simulink model "InteractiveArmModel_R2021a_v1"  (R2021a)
settings: Solver=ode4  StartTime=0.0  StopTime=3000  FixedStep=1/150  MaxStep=1/50  MinStep=1/200  RelTol=1e-5  AbsTol=1e-6  EnableMultiTasking=on
model workspace (MAT data in the model file):
  MaxEccentricFlexor = 0.5
  PoleZ = 0.85
  SampleTime = 0.05
  musNoise = 0
  musNoiseLevel : Simulink.Parameter (value not decoded)
libraries: simulink x1
(part 3 of 3)

== system InteractiveArmModel_R2021a_v1/Trial Start//Stop//Increment Control/Flag for What Phase Trial is In/If Action Subsystem6 ==
  In1 : Inport
  Action Port : ActionPort  ActionPortLabel=elseif(u2 == 0)
  Out1 : Outport
  wires:
  In1/1 -> Out1/1

== system InteractiveArmModel_R2021a_v1/Trial Start//Stop//Increment Control/Flag for What Phase Trial is In/If Action Subsystem7 ==
  In1 : Inport
  Action Port : ActionPort  ActionPortLabel=else
  Out1 : Outport
  wires:
  In1/1 -> Out1/1

== system InteractiveArmModel_R2021a_v1/Trial Start//Stop//Increment Control/Stop Criteria Flag Control (Between Trials)/If Action Subsystem3 ==
  In1 : Inport
  Action Port : ActionPort  ActionPortLabel=if(u1 == 0)
  Out1 : Outport
  wires:
  In1/1 -> Out1/1

== system InteractiveArmModel_R2021a_v1/Trial Start//Stop//Increment Control/Stop Criteria Flag Control (Between Trials)/If Action Subsystem4 ==
  In1 : Inport
  Action Port : ActionPort  ActionPortLabel=else
  Out1 : Outport
  wires:
  In1/1 -> Out1/1

== system InteractiveArmModel_R2021a_v1/Trial Start//Stop//Increment Control/Subsystem/If Action Subsystem ==
  In1 : Inport
  Action Port : ActionPort  ActionPortLabel=if(u1 == 0)
  Out1 : Outport
  wires:
  In1/1 -> Out1/1

== system InteractiveArmModel_R2021a_v1/Trial Start//Stop//Increment Control/Subsystem2/If Action Subsystem1 ==
  In1 : Inport
  Action Port : ActionPort  ActionPortLabel=if(u1 < 0.01)
  Out1 : Outport
  wires:
  In1/1 -> Out1/1

== system InteractiveArmModel_R2021a_v1/Trial Start//Stop//Increment Control/Subsystem2/If Action Subsystem2 ==
  In1 : Inport
  Action Port : ActionPort  ActionPortLabel=else
  Out1 : Outport
  wires:
  In1/1 -> Out1/1

== system InteractiveArmModel_R2021a_v1/While Loop (Main Simulation Code)/Integrator 1/Integrater ==
  Accel : Inport
  Add : Sum
  Delay : Delay  DelayLength=1  InitialCondition=0
  Delay1 : Delay  DelayLength=1  InitialCondition=0
  Digital Clock : DigitalClock  SampleTime=-1
  Product : Product
  Subtract : Sum  Inputs=+-
  Vel : Outport
  wires:
  Accel/1 -> Product/2
  Subtract/1 -> Product/1
  Product/1 -> Add/1
  Add/1 -> Delay/1
  Delay/1 -> Vel/1, Add/2
  Digital Clock/1 -> Subtract/1, Delay1/1
  Delay1/1 -> Subtract/2

== system InteractiveArmModel_R2021a_v1/While Loop (Main Simulation Code)/Integrator 1/Reset ==
  Reset : Inport
  " Accel" : Inport  Port=2
  If : If  IfExpression=u1 == 0  ShowElse=off
  If Action Subsystem : Subsystem  TreatAsAtomicUnit=on
  Subtract : Sum  Inputs=+-
  Accel : Outport
  wires:
  Reset/1 -> If/1
  If/1 -> If Action Subsystem/Action
  Subtract/1 -> Accel/1
  " Accel"/1 -> Subtract/1, If Action Subsystem/1(In1)
  If Action Subsystem/1(Out1) -> Subtract/2

== system InteractiveArmModel_R2021a_v1/While Loop (Main Simulation Code)/Integrator 1/Reset2 ==
  Reset : Inport
  VelIn : Inport  Port=2
  If : If  IfExpression=u1 == 0  ShowElse=off
  If Action Subsystem : Subsystem  TreatAsAtomicUnit=on
  Subtract : Sum  Inputs=+-
  VelOut : Outport
  wires:
  Reset/1 -> If/1
  If/1 -> If Action Subsystem/Action
  Subtract/1 -> VelOut/1
  VelIn/1 -> Subtract/1, If Action Subsystem/1(In1)
  If Action Subsystem/1(Out1) -> Subtract/2

== system InteractiveArmModel_R2021a_v1/While Loop (Main Simulation Code)/Integrator 2/Integrater 1 ==
  VelIn : Inport
  Add : Sum
  Delay : Delay  DelayLength=1  InitialCondition=0
  Delay1 : Delay  DelayLength=1  InitialCondition=0
  Digital Clock : DigitalClock  SampleTime=-1
  Product : Product
  Subtract : Sum  Inputs=+-
  PosOut : Outport
  wires:
  VelIn/1 -> Product/2
  Subtract/1 -> Product/1
  Product/1 -> Add/1
  Add/1 -> Delay/1
  Delay/1 -> PosOut/1, Add/2
  Digital Clock/1 -> Subtract/1, Delay1/1
  Delay1/1 -> Subtract/2

== system InteractiveArmModel_R2021a_v1/While Loop (Main Simulation Code)/Integrator 2/Reset2 ==
  Reset : Inport
  PosIn : Inport  Port=2
  If : If  IfExpression=u1 == 0  ShowElse=off
  If Action Subsystem : Subsystem  TreatAsAtomicUnit=on
  Subtract : Sum  Inputs=+-
  PosOut : Outport
  wires:
  Reset/1 -> If/1
  If/1 -> If Action Subsystem/Action
  Subtract/1 -> PosOut/1
  PosIn/1 -> Subtract/1, If Action Subsystem/1(In1)
  If Action Subsystem/1(Out1) -> Subtract/2

== system InteractiveArmModel_R2021a_v1/While Loop (Main Simulation Code)/Muscle Models/Add Noise to Keyboard // Mouse Control Input Types ==
  In1 : Inport
  Add1 : Sum
  Add2 : Sum
  Demux2 : Demux  Outputs=2
  If : If  IfExpression=u1 > 0.01
  If Action Subsystem : Subsystem  TreatAsAtomicUnit=on
  If Action Subsystem1 : Subsystem  TreatAsAtomicUnit=on
  If Action Subsystem2 : Subsystem  TreatAsAtomicUnit=on
  If Action Subsystem3 : Subsystem  TreatAsAtomicUnit=on
  If2 : If  IfExpression=u1 > 0.01
  Merge : Merge
  Merge2 : Merge
  Mux1 : Mux  Inputs=2
  Random Number : RandomNumber  Variance=musNoise
  Random Number1 : RandomNumber  Variance=musNoise
  Scope : Scope
  Out1 : Outport
  wires:
  If Action Subsystem2/1(Out1) -> Merge2/1
  If/2 -> If Action Subsystem1/Action
  Demux2/1 -> If/1, If Action Subsystem1/1(In1), Add1/1
  Random Number/1 -> Scope/1, Add1/2
  Demux2/2 -> If2/1, Add2/1, If Action Subsystem3/1(In1)
  Merge/1 -> Mux1/1
  Add1/1 -> If Action Subsystem/1(In1)
  Merge2/1 -> Mux1/2
  Add2/1 -> If Action Subsystem2/1(In1)
  If Action Subsystem3/1(Out1) -> Merge2/2
  If2/2 -> If Action Subsystem3/Action
  If2/1 -> If Action Subsystem2/Action
  If Action Subsystem1/1(Out1) -> Merge/2
  Random Number1/1 -> Add2/2
  If/1 -> If Action Subsystem/Action
  If Action Subsystem/1(Out1) -> Merge/1
  In1/1 -> Demux2/1
  Mux1/1 -> Out1/1

== system InteractiveArmModel_R2021a_v1/While Loop (Main Simulation Code)/Muscle Models/EMG Calibration1 ==
  stimulation(flex+Ext) : Inport
  Demux : Demux  Outputs=2
  Divide : Product  Inputs=*/
  Divide1 : Product  Inputs=*/
  Maxima Ext : Constant  Value=980
  Maxima Flex : Constant  Value=980
  Minima Ext : Constant  Value=80
  Minima Flex : Constant  Value=50
  Mux : Mux  Inputs=2
  Saturation : Saturate  UpperLimit=1  LowerLimit=0
  Saturation1 : Saturate  UpperLimit=1  LowerLimit=0
  Subtract{1..4} (4 alike) : Sum  Inputs=+-
  Excitation (Range: 0-1) : Outport
  wires:
  Subtract3/1 -> Divide/2
  Subtract4/1 -> Divide/1
  Divide/1 -> Saturation/1
  Minima Flex/1 -> Subtract3/2, Subtract4/2
  Maxima Flex/1 -> Subtract3/1
  stimulation(flex+Ext)/1 -> Demux/1
  Demux/1 -> Subtract4/1  "FLEX"
  Demux/2 -> Subtract2/1  "EXT"
  Saturation1/1 -> Mux/2
  Subtract2/1 -> Divide1/1
  Divide1/1 -> Saturation1/1
  Minima Ext/1 -> Subtract1/2, Subtract2/2
  Subtract1/1 -> Divide1/2
  Maxima Ext/1 -> Subtract1/1
  Mux/1 -> Excitation (Range: 0-1)/1
  Saturation/1 -> Mux/1

== system InteractiveArmModel_R2021a_v1/While Loop (Main Simulation Code)/Muscle Models/EMG Control ==
  stimulation(flex+Ext) : Inport
  Action Port : ActionPort  ActionPortLabel=elseif( u1 == 2)
  Out1 : Outport
  wires:
  stimulation(flex+Ext)/1 -> Out1/1

== system InteractiveArmModel_R2021a_v1/While Loop (Main Simulation Code)/Muscle Models/Extensor Muscle Mechanics ==
  note: Activation
  "Excitation Extensor " : Inport
  IC : Inport  Port=2
  LMT Extensor : Inport  Port=3
  ModelAge : Inport  Port=4
  Bounds Checks : Subsystem
  Constant13 : Constant
  Delay : Delay  DelayLength=1  InitialCondition=0
  Force-Velocity Relation : FunctionCaller  FunctionPrototype=[vSEE,dPdt,vCE] = Muscle_Mechanics_Functions.FVR(FP,Vmt,p,flexext,activation,ModelStrength)  InputArgumentSpecifications=<Enter example>  OutputArgumentSpecifications=<Enter example>
  Function Caller : FunctionCaller  FunctionPrototype=ActivationChange = Muscle_Mechanics_Functions.ExciteAct(IC,Excitation,WhichMus,PreviousAct)  InputArgumentSpecifications=<Enter example>  OutputArgumentSpecifications=<Enter example>
  Function Caller1 : FunctionCaller  FunctionPrototype=[FP,LCC] = Muscle_Mechanics_Functions.FLR(Lmt,L_SEE,Activation,FlexExt,ModelStrength)  InputArgumentSpecifications=<Enter example>  OutputArgumentSpecifications=<Enter example>
  Function Caller3 : FunctionCaller  FunctionPrototype=L_SEE = Muscle_Mechanics_Functions.LSEE(P,FlexOrExtMus,ModelStrength)  InputArgumentSpecifications=<Enter example>  OutputArgumentSpecifications=<Enter example>
  IEEE Double Discrete Time Filtered Derivative : DiscreteFilter  Numerator=(1-PoleZ)*[1 -1]  Denominator=SampleTime*[1 -PoleZ]
  Integrate Act Change : Subsystem
  Reset : Subsystem
  Subsystem : Subsystem
  To Workspace1 : ToWorkspace  VariableName=activationExt  SaveFormat=Timeseries  SampleTime=-1
  To Workspace2 : ToWorkspace  VariableName=forcePotentialExt  SaveFormat=Timeseries  SampleTime=-1
  To Workspace3 : ToWorkspace  VariableName=lengthCC_Ext  SaveFormat=Timeseries  SampleTime=-1
  To Workspace4 : ToWorkspace  VariableName=musVelExt  SaveFormat=Timeseries  SampleTime=-1
  To Workspace5 : ToWorkspace  VariableName=velSEE_Ext  SaveFormat=Timeseries  SampleTime=-1
  To Workspace6 : ToWorkspace  VariableName=lenSEE_Ext  SaveFormat=Timeseries  SampleTime=-1
  To Workspace7 : ToWorkspace  VariableName=musLenExt  SaveFormat=Timeseries  SampleTime=-1
  To Workspace8 : ToWorkspace  VariableName=velCE_Ext  SaveFormat=Timeseries  SampleTime=-1
  P Extenasor : Outport
  wires:
  Constant13/1 -> Function Caller3/2, Function Caller1/4, Force-Velocity Relation/4, Function Caller/3
  Function Caller3/1 -> To Workspace6/1, Function Caller1/2  "Ext LSEE"
  Function Caller1/1 -> To Workspace2/1, Force-Velocity Relation/1  "Ext FP"
  Function Caller1/2 -> To Workspace3/1  "Ext LCC"
  LMT Extensor/1 -> IEEE Double Discrete Time Filtered Derivative/1, To Workspace7/1, Function Caller1/1  "Lmt"
  Subsystem/1(Force) -> Reset/2(" ")  "P Extenasor"
  Reset/1("Force ") -> Bounds Checks/2("Force ")
  Force-Velocity Relation/2 -> Subsystem/1(dp/dt)
  Force-Velocity Relation/1 -> To Workspace5/1  "dP/dt Extensor"
  Force-Velocity Relation/3 -> To Workspace8/1
  "Excitation Extensor "/1 -> Function Caller/2
  Delay/1 -> Function Caller/4
  IC/1 -> Function Caller/1, Reset/1(1), Integrate Act Change/1(IC)
  Integrate Act Change/1(Activation) -> Function Caller1/3, Force-Velocity Relation/5, Delay/1, Bounds Checks/1(Activation), To Workspace1/1
  Function Caller/1 -> Integrate Act Change/2(In2)
  Bounds Checks/1(P Flexor) -> P Extenasor/1, Function Caller3/1, Force-Velocity Relation/3
  ModelAge/1 -> Bounds Checks/3(ModelAge), Force-Velocity Relation/6, Function Caller1/5, Function Caller3/3
  IEEE Double Discrete Time Filtered Derivative/1 -> Force-Velocity Relation/2, To Workspace4/1  "Discrete-Time Filtered Derivative"

== system InteractiveArmModel_R2021a_v1/While Loop (Main Simulation Code)/Muscle Models/Flexor Muscle Mechanics ==
  note: From "Fixed-Point Derivatives" simulink example.
      | https://www.mathworks.com/help/fixedpoint/ug/fixed-point-derivatives.html
  note: Activation
  ExcitationFlexor : Inport
  IC : Inport  Port=2
  LmtFlexor : Inport  Port=3
  ModelAge : Inport  Port=4
  Bounds Checks : Subsystem
  Delay : Delay  DelayLength=1  InitialCondition=0
  FlexorOrExtensorConstant : Constant  Value=2
  Force-Extension Relation : FunctionCaller  FunctionPrototype=L_SEE = Muscle_Mechanics_Functions.LSEE(P,FlexOrExtMus,ModelStrength)  InputArgumentSpecifications=<Enter example>  OutputArgumentSpecifications=<Enter example>
  Force-Length Relationship : FunctionCaller  FunctionPrototype=[FP,LCC] = Muscle_Mechanics_Functions.FLR(Lmt,L_SEE,Activation,FlexExt,ModelStrength)  InputArgumentSpecifications=<Enter example>  OutputArgumentSpecifications=<Enter example>
  Force-Velocity Relationship : FunctionCaller  FunctionPrototype=[vSEE,dPdt,vCE] = Muscle_Mechanics_Functions.FVR(FP,Vmt,p,flexext,activation,ModelStrength)  InputArgumentSpecifications=<Enter example>  OutputArgumentSpecifications=<Enter example>
  Function Caller1 : FunctionCaller  FunctionPrototype=ActivationChange = Muscle_Mechanics_Functions.ExciteAct(IC,Excitation,WhichMus,PreviousAct)  InputArgumentSpecifications=<Enter example>  OutputArgumentSpecifications=<Enter example>
  IEEE Double Discrete Time Filtered Derivative : DiscreteFilter  Numerator=(1-PoleZ)*[1 -1]  Denominator=SampleTime*[1 -PoleZ]
  Integrate Act Change : Subsystem
  Integrater : Subsystem
  Reset : Subsystem
  To Workspace10 : ToWorkspace  VariableName=velCE_Flex1  SaveFormat=Timeseries  SampleTime=-1
  To Workspace3 : ToWorkspace  VariableName=activationFlex1  SaveFormat=Timeseries  SampleTime=-1
  To Workspace4 : ToWorkspace  VariableName=forcePotentialFlex1  SaveFormat=Timeseries  SampleTime=-1
  To Workspace5 : ToWorkspace  VariableName=lengthCC_Flex1  SaveFormat=Timeseries  SampleTime=-1
  To Workspace6 : ToWorkspace  VariableName=musVelFlex1  SaveFormat=Timeseries  SampleTime=-1
  To Workspace7 : ToWorkspace  VariableName=lenSEE_Flex1  SaveFormat=Timeseries  SampleTime=-1
  To Workspace8 : ToWorkspace  VariableName=velSEE_Flex1  SaveFormat=Timeseries  SampleTime=-1
  To Workspace9 : ToWorkspace  VariableName=musLenFlex1  SaveFormat=Timeseries  SampleTime=-1
  P Flexor : Outport
  wires:
  FlexorOrExtensorConstant/1 -> Function Caller1/3, Force-Extension Relation/2, Force-Length Relationship/4, Force-Velocity Relationship/4
  IEEE Double Discrete Time Filtered Derivative/1 -> To Workspace6/1, Force-Velocity Relationship/2  "Discrete-Time Filtered Derivative"
  Force-Length Relationship/2 -> To Workspace5/1  "Flex LCC"
  Bounds Checks/1(P Flexor) -> Force-Extension Relation/1, Force-Velocity Relationship/3, P Flexor/1
  Integrater/1(1) -> Reset/2(" ")  "P Extenasor"
  Integrate Act Change/1(Out1) -> Force-Velocity Relationship/5, Delay/1, Force-Length Relationship/3, Bounds Checks/1(Activation), To Workspace3/1
  Reset/1("Force ") -> Bounds Checks/2("Force ")
  ModelAge/1 -> Bounds Checks/3(ModelAge), Force-Velocity Relationship/6, Force-Length Relationship/5, Force-Extension Relation/3
  LmtFlexor/1 -> IEEE Double Discrete Time Filtered Derivative/1, To Workspace9/1, Force-Length Relationship/1
  IC/1 -> Integrate Act Change/1(IC), Function Caller1/1, Reset/1(1)
  Force-Length Relationship/1 -> To Workspace4/1, Force-Velocity Relationship/1  "Flex FP"
  Force-Velocity Relationship/2 -> Integrater/1(In1)
  Force-Extension Relation/1 -> To Workspace7/1, Force-Length Relationship/2  "Flex LSEE"
  Force-Velocity Relationship/1 -> To Workspace8/1  "dP/dt"
  Delay/1 -> Function Caller1/4
  ExcitationFlexor/1 -> Function Caller1/2
  Function Caller1/1 -> Integrate Act Change/2(In2)
  Force-Velocity Relationship/3 -> To Workspace10/1

== system InteractiveArmModel_R2021a_v1/While Loop (Main Simulation Code)/Muscle Models/Keyboard Control ==
  stimulation(flex+Ext) : Inport
  Action Port : ActionPort  ActionPortLabel=if(u1 == 0)
  Out1 : Outport
  wires:
  stimulation(flex+Ext)/1 -> Out1/1

== system InteractiveArmModel_R2021a_v1/While Loop (Main Simulation Code)/Muscle Models/Mouse Control ==
  stimulation(flex+Ext) : Inport
  Action Port : ActionPort  ActionPortLabel=elseif(u1 == 1)
  Out1 : Outport
  wires:
  stimulation(flex+Ext)/1 -> Out1/1

== system InteractiveArmModel_R2021a_v1/While Loop (Main Simulation Code)/Musculoskeletal Geometry/LMT Extensor ==
  angle (r) : Inport
  Lower Arm length (m) : Inport  Port=2
  upper arm length (m) : Inport  Port=3
  Add : Sum
  Constant : Constant  Value=0.1
  Constant1 : Constant  Value=0.9
  Cos : Trigonometry  Operator=cos
  Math Function : Math  Operator=square  SaturateOnIntegerOverflow=on
  Math Function1 : Math  Operator=square  SaturateOnIntegerOverflow=on
  Product{1..4} (4 alike) : Product
  Sqrt : Sqrt  SaturateOnIntegerOverflow=on
  Subtract : Sum  Inputs=+-
  Trigonometric Function : Trigonometry
  Lmt Extensor (m) : Outport
  Proximal Ext Muscle attachment (m),x : Outport  Port=2
  Distal Ext Muscle Attachment (m) ,x : Outport  Port=3
  Distal Ext Muscle Attachment (m) ,y : Outport  Port=4
  wires:
  Subtract/1 -> Math Function/1
  Math Function/1 -> Add/2
  angle (r)/1 -> Trigonometric Function/1, Cos/1
  Constant1/1 -> Product1/2
  Add/1 -> Sqrt/1
  Product4/1 -> Distal Ext Muscle Attachment (m) ,y/1, Math Function1/1
  Product1/1 -> Proximal Ext Muscle attachment (m),x/1, Subtract/2
  Product3/1 -> Distal Ext Muscle Attachment (m) ,x/1, Subtract/1
  Product2/1 -> Product3/2, Product4/2
  Cos/1 -> Product3/1
  Math Function1/1 -> Add/1
  Constant/1 -> Product2/1
  upper arm length (m)/1 -> Product1/1
  Lower Arm length (m)/1 -> Product2/2
  Sqrt/1 -> Lmt Extensor (m)/1
  Trigonometric Function/1 -> Product4/1

== system InteractiveArmModel_R2021a_v1/While Loop (Main Simulation Code)/Musculoskeletal Geometry/LMT Flexor ==
  angle (r) : Inport
  lower arm length (m) : Inport  Port=2
  upper arm length (m) : Inport  Port=3
  Add : Sum
  Add1 : Sum
  Constant : Constant  Value=0.1
  Constant1 : Constant  Value=0.9
  Cos : Trigonometry  Operator=cos
  Math Function : Math  Operator=square  SaturateOnIntegerOverflow=on
  Math Function1 : Math  Operator=square  SaturateOnIntegerOverflow=on
  Product{1..4} (4 alike) : Product
  Sqrt : Sqrt  SaturateOnIntegerOverflow=on
  Trigonometric Function : Trigonometry
  Lmt Flexor (m) : Outport
  "Proximal Flex muscle Attachment (m), x " : Outport  Port=2
  "Distal Flex muscle Attachment (m), x" : Outport  Port=3
  "Distal Flex muscle Attachment (m), y " : Outport  Port=4
  wires:
  Add1/1 -> Math Function/1
  Math Function/1 -> Add/2
  angle (r)/1 -> Trigonometric Function/1, Cos/1
  Constant1/1 -> Product1/2
  Add/1 -> Sqrt/1
  Product4/1 -> "Distal Flex muscle Attachment (m), y "/1, Math Function1/1
  Product1/1 -> Add1/2, "Proximal Flex muscle Attachment (m), x "/1
  Product3/1 -> Add1/1, "Distal Flex muscle Attachment (m), x"/1
  Product2/1 -> Product4/2, Product3/2
  Cos/1 -> Product3/1
  Math Function1/1 -> Add/1
  Constant/1 -> Product2/1
  upper arm length (m)/1 -> Product1/1
  lower arm length (m)/1 -> Product2/2
  Sqrt/1 -> Lmt Flexor (m)/1
  Trigonometric Function/1 -> Product4/1

== system InteractiveArmModel_R2021a_v1/While Loop (Main Simulation Code)/Musculoskeletal Geometry/MA Extensor ==
  angle (radians) : Inport
  Lmt Extensor (m) : Inport  Port=2
  lower arm length (m) : Inport  Port=3
  Upper arm length (m) : Inport  Port=4
  Asin : Trigonometry  Operator=asin
  Constant2 : Constant  Value=-1
  Divide : Product  Inputs=*/
  Location of Muscle Insertion : FunctionCaller  FunctionPrototype=y = Constants.insertLoc()  OutputArgumentSpecifications=<Enter example>
  Location of Muscle Origin : FunctionCaller  FunctionPrototype=y = Constants.originLoc()  OutputArgumentSpecifications=<Enter example>
  Product : Product  Inputs=3
  Product1 : Product  Inputs=3
  Product2 : Product
  Trigonometric Function : Trigonometry
  Trigonometric Function1 : Trigonometry
  Extensor Moment arm (m) : Outport
  wires:
  Product1/1 -> Divide/1
  Trigonometric Function1/1 -> Product/2
  Upper arm length (m)/1 -> Product/3
  Trigonometric Function/1 -> Product1/1
  Divide/1 -> Asin/1
  lower arm length (m)/1 -> Product1/3
  Location of Muscle Insertion/1 -> Product1/2
  Asin/1 -> Trigonometric Function1/1
  Lmt Extensor (m)/1 -> Divide/2
  angle (radians)/1 -> Trigonometric Function/1
  Product/1 -> Extensor Moment arm (m)/1
  Constant2/1 -> Product2/1
  Location of Muscle Origin/1 -> Product2/2
  Product2/1 -> Product/1

== system InteractiveArmModel_R2021a_v1/While Loop (Main Simulation Code)/Musculoskeletal Geometry/MA Flexor ==
  note: The distance from the elbow to the origin of the flexors and extensors is 90% of the length of the upper arm (starting from the elbow and going proximal).
  note: The distance from the elbow to the insertion of the flexor and extensors is 10% of the length of the lower arm (starting from the elbow and going distal).
  note: Location of flexor/ext origin is 10% of distance from shoulder to elbow (going distal from shoulder).
  angle (radians) : Inport
  Lmt Extensor (m) : Inport  Port=2
  Lower arm length (m) : Inport  Port=3
  Upper arm length (m) : Inport  Port=4
  Asin : Trigonometry  Operator=asin
  Divide : Product  Inputs=*/
  Location of Muscle Insertion : FunctionCaller  FunctionPrototype=y = Constants.insertLoc()  OutputArgumentSpecifications=<Enter example>
  Location of Muscle Origin : FunctionCaller  FunctionPrototype=y = Constants.originLoc()  OutputArgumentSpecifications=<Enter example>
  Product : Product  Inputs=3
  Product1 : Product  Inputs=3
  Trigonometric Function : Trigonometry
  Trigonometric Function1 : Trigonometry
  Flexor moment arm (m) : Outport
  wires:
  Product1/1 -> Divide/1
  Trigonometric Function1/1 -> Product/2
  Upper arm length (m)/1 -> Product/3
  Trigonometric Function/1 -> Product1/1
  Divide/1 -> Asin/1
  Lower arm length (m)/1 -> Product1/3
  Asin/1 -> Trigonometric Function1/1
  Lmt Extensor (m)/1 -> Divide/2
  angle (radians)/1 -> Trigonometric Function/1
  Product/1 -> Flexor moment arm (m)/1
  Location of Muscle Origin/1 -> Product/1
  Location of Muscle Insertion/1 -> Product1/2

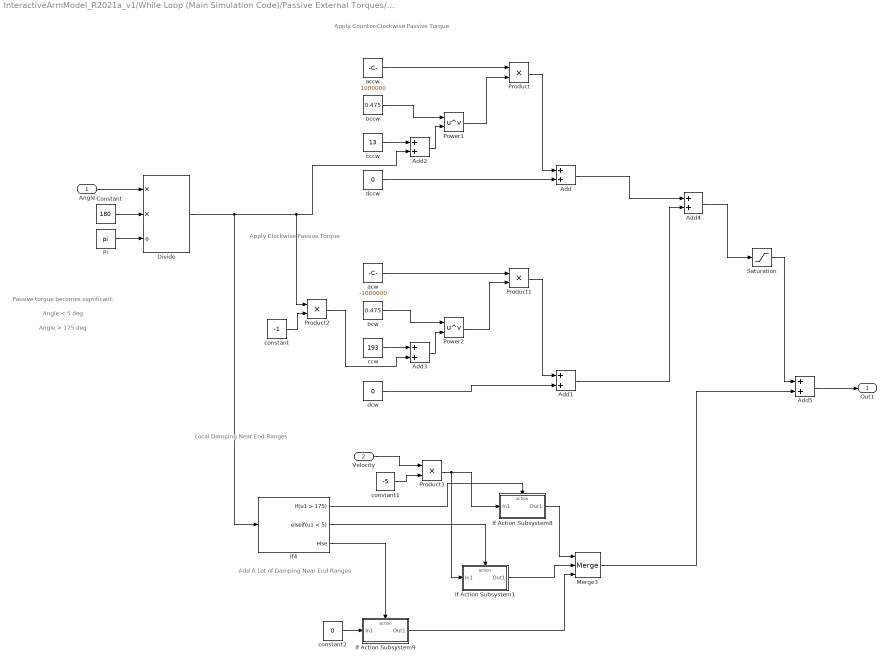
== system InteractiveArmModel_R2021a_v1/While Loop (Main Simulation Code)/Passive External Torques/Passive torque ==
  note: Apply Clockwise Passive Torque
  note: Apply Counter-Clockwise Passive Torque
  note: Local Damping Near End Ranges
  note: Add A Lot of Damping Near End Ranges
  note: Angle > 175 deg
  note: Angle < 5 deg
  note: Passive torque becomes significant:
  Angle : Inport
  Velocity : Inport  Port=2
  Add{,1..5} (6 alike) : Sum
  Constant : Constant  Value=180
  Divide : Product  Inputs=**/
  If Action Subsystem1 : Subsystem  TreatAsAtomicUnit=on
  If Action Subsystem8 : Subsystem  TreatAsAtomicUnit=on
  If Action Subsystem9 : Subsystem  TreatAsAtomicUnit=on
  If4 : If  IfExpression=u1 > 175  ElseIfExpressions=u1 < 5
  Merge3 : Merge  Inputs=3
  Pi : Constant  Value=pi  OutDataTypeStr=Inherit: Inherit via back propagation
  Power1 : Math  Operator=pow  SaturateOnIntegerOverflow=on
  Power2 : Math  Operator=pow  SaturateOnIntegerOverflow=on
  Product{,1..3} (4 alike) : Product
  Saturation : Saturate  UpperLimit=100  LowerLimit=-100
  accw : Constant  Value=1000000
  acw : Constant  Value=-1000000
  bccw : Constant  Value=0.475
  bcw : Constant  Value=0.475
  cccw : Constant  Value=13
  ccw : Constant  Value=193
  constant : Constant  Value=-1
  constant1 : Constant  Value=-5
  constant2 : Constant  Value=0
  dccw : Constant  Value=0
  dcw : Constant  Value=0
  Out1 : Outport
  wires:
  Add2/1 -> Power1/2
  Product1/1 -> Add1/1
  Power2/1 -> Product1/2
  constant/1 -> Product2/2
  Add/1 -> Add4/1
  Divide/1 -> If4/1, Product2/1, Add2/2
  accw/1 -> Product/1
  Power1/1 -> Product/2
  acw/1 -> Product1/1
  Add3/1 -> Power2/2
  bcw/1 -> Power2/1
  Product2/1 -> Add3/2
  dcw/1 -> Add1/2
  dccw/1 -> Add/2
  bccw/1 -> Power1/1
  Product/1 -> Add/1
  cccw/1 -> Add2/1
  ccw/1 -> Add3/1
  Angle/1 -> Divide/1
  Constant/1 -> Divide/2
  Pi/1 -> Divide/3
  Add1/1 -> Add4/2
  Product3/1 -> If Action Subsystem1/1(In1), If Action Subsystem8/1(In1)
  If4/1 -> If Action Subsystem8/Action
  If Action Subsystem8/1(Out1) -> Merge3/1
  If4/3 -> If Action Subsystem9/Action
  If Action Subsystem9/1(Out1) -> Merge3/3
  Velocity/1 -> Product3/1
  constant1/1 -> Product3/2
  constant2/1 -> If Action Subsystem9/1(In1)
  If4/2 -> If Action Subsystem1/Action
  If Action Subsystem1/1(Out1) -> Merge3/2
  Merge3/1 -> Add5/2
  Add5/1 -> Out1/1
  Add4/1 -> Saturation/1
  Saturation/1 -> Add5/1

== system InteractiveArmModel_R2021a_v1/Muscle_Mechanics_Functions/Contractile Element Force-Length Relation/S1, S2, S3 calculation/S1 ==
  note: C
  note: L
  In1 : Inport
  In2 : Inport  Port=2
  Constant : Constant
  Math Function : Math  Operator=square  SaturateOnIntegerOverflow=on
  Product : Product
  Subtract : Sum  Inputs=+-
  Out1 : Outport
  wires:
  In1/1 -> Math Function/1
  Math Function/1 -> Product/1
  In2/1 -> Product/2
  Product/1 -> Subtract/2
  Constant/1 -> Subtract/1
  Subtract/1 -> Out1/1

== system InteractiveArmModel_R2021a_v1/Muscle_Mechanics_Functions/Contractile Element Force-Length Relation/S1, S2, S3 calculation/S2 ==
  note: C
  note: L
  In1 : Inport
  In2 : Inport  Port=2
  In3 : Inport  Port=3
  Constant : Constant  Value=-2
  Divide : Product  Inputs=*/
  Exp : Math  SaturateOnIntegerOverflow=on
  Math Function : Math  Operator=square  SaturateOnIntegerOverflow=on
  Product : Product  Inputs=3
  Out1 : Outport
  wires:
  In1/1 -> Math Function/1
  In2/1 -> Product/2
  Math Function/1 -> Product/1
  Constant/1 -> Product/3
  Product/1 -> Divide/1
  In3/1 -> Divide/2  "S1"
  Divide/1 -> Exp/1
  Exp/1 -> Out1/1

== system InteractiveArmModel_R2021a_v1/Muscle_Mechanics_Functions/Contractile Element Force-Length Relation/S1, S2, S3 calculation/S3 ==
  note: C
  note: L
  In1 : Inport
  In2 : Inport  Port=2
  S1 : Inport  Port=3
  normalised CC length : Inport  Port=4
  Constant : Constant
  Constant1 : Constant  Value=-2
  Divide : Product  Inputs=*/
  Exp : Math  SaturateOnIntegerOverflow=on
  Product : Product
  Product1 : Product  Inputs=3
  Scope : Scope  NumInputPorts=2
  Subtract : Sum  Inputs=+-
  Out1 : Outport
  Out2 : Outport  Port=2
  wires:
  normalised CC length/1 -> Subtract/1
  Constant/1 -> Subtract/2
  Subtract/1 -> Product/2
  In1/1 -> Product/1
  In2/1 -> Product1/1
  Constant1/1 -> Product1/2
  Product/1 -> Product1/3
  Product1/1 -> Divide/1
  S1/1 -> Divide/2
  Divide/1 -> Scope/1, Out2/1, Exp/1
  Exp/1 -> Scope/2, Out1/1

== system InteractiveArmModel_R2021a_v1/Muscle_Mechanics_Functions/Contractile Element Force-Length Relation/S1, S2, S3 calculation/S3 for condition 2 ==
  In1 : Inport
  Constant : Constant  Value=-1
  Exp : Math  SaturateOnIntegerOverflow=on
  Product : Product
  Out1 : Outport
  wires:
  In1/1 -> Product/2
  Constant/1 -> Product/1
  Product/1 -> Exp/1
  Exp/1 -> Out1/1

== system InteractiveArmModel_R2021a_v1/While Loop (Main Simulation Code)/Integrator 1/Reset/If Action Subsystem ==
  In1 : Inport
  Action Port : ActionPort  ActionPortLabel=if(u1 == 0)
  Out1 : Outport
  wires:
  In1/1 -> Out1/1

== system InteractiveArmModel_R2021a_v1/While Loop (Main Simulation Code)/Integrator 1/Reset2/If Action Subsystem ==
  In1 : Inport
  Action Port : ActionPort  ActionPortLabel=if(u1 == 0)
  Out1 : Outport
  wires:
  In1/1 -> Out1/1

== system InteractiveArmModel_R2021a_v1/While Loop (Main Simulation Code)/Integrator 2/Reset2/If Action Subsystem ==
  In1 : Inport
  Action Port : ActionPort  ActionPortLabel=if(u1 == 0)
  Out1 : Outport
  wires:
  In1/1 -> Out1/1

== system InteractiveArmModel_R2021a_v1/While Loop (Main Simulation Code)/Muscle Models/Add Noise to Keyboard // Mouse Control Input Types/If Action Subsystem ==
  In1 : Inport
  Action Port : ActionPort  ActionPortLabel=if(u1 > 0.01)
  Out1 : Outport
  wires:
  In1/1 -> Out1/1

== system InteractiveArmModel_R2021a_v1/While Loop (Main Simulation Code)/Muscle Models/Add Noise to Keyboard // Mouse Control Input Types/If Action Subsystem1 ==
  In1 : Inport
  Action Port : ActionPort  ActionPortLabel=else
  Out1 : Outport
  wires:
  In1/1 -> Out1/1

== system InteractiveArmModel_R2021a_v1/While Loop (Main Simulation Code)/Muscle Models/Add Noise to Keyboard // Mouse Control Input Types/If Action Subsystem2 ==
  In1 : Inport
  Action Port : ActionPort  ActionPortLabel=if(u1 > 0.01)
  Out1 : Outport
  wires:
  In1/1 -> Out1/1

== system InteractiveArmModel_R2021a_v1/While Loop (Main Simulation Code)/Muscle Models/Add Noise to Keyboard // Mouse Control Input Types/If Action Subsystem3 ==
  In1 : Inport
  Action Port : ActionPort  ActionPortLabel=else
  Out1 : Outport
  wires:
  In1/1 -> Out1/1

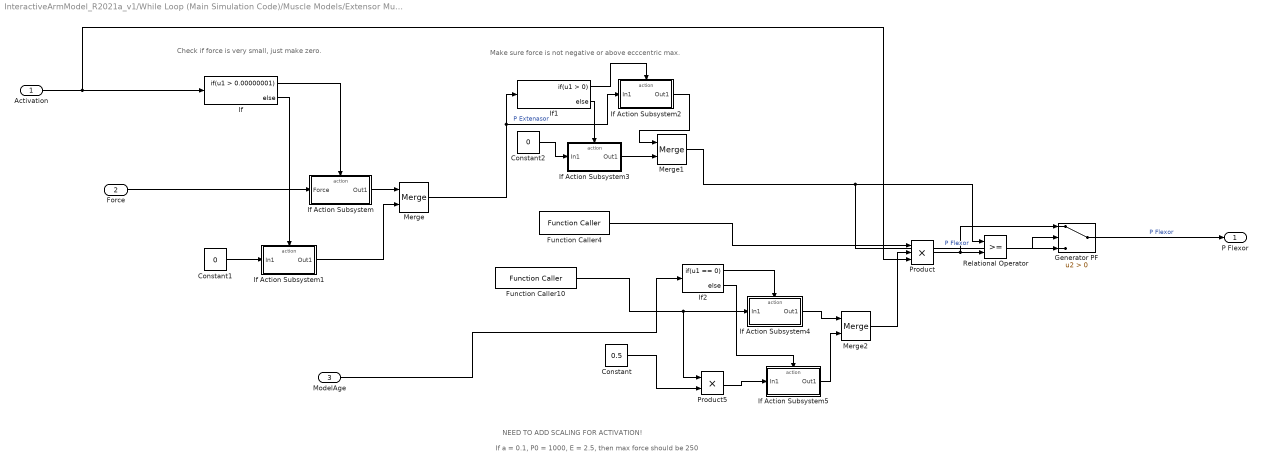
== system InteractiveArmModel_R2021a_v1/While Loop (Main Simulation Code)/Muscle Models/Extensor Muscle Mechanics/Bounds Checks ==
  note: If a = 0.1, P0 = 1000, E = 2.5, then max force should be 250
  note: NEED TO ADD SCALING FOR ACTIVATION!
  note: Check if force is very small, just make zero.
  note: Make sure force is not negative or above ecccentric max.
  Activation : Inport
  "Force " : Inport  Port=2
  ModelAge : Inport  Port=3
  Constant : Constant  Value=0.5
  Constant1 : Constant  Value=0
  Constant2 : Constant  Value=0
  Function Caller10 : FunctionCaller  FunctionPrototype=y = Constants.P0F()  InputArgumentSpecifications=<Enter example>  OutputArgumentSpecifications=<Enter example>
  Function Caller4 : FunctionCaller  FunctionPrototype=y = Constants.EF()  InputArgumentSpecifications=<Enter example>  OutputArgumentSpecifications=<Enter example>
  Generator PF : Switch  Criteria=u2 > Threshold
  If : If  IfExpression=u1 > 0.00000001
  If Action Subsystem : Subsystem  TreatAsAtomicUnit=on
  If Action Subsystem1 : Subsystem  TreatAsAtomicUnit=on
  If Action Subsystem2 : Subsystem  TreatAsAtomicUnit=on
  If Action Subsystem3 : Subsystem  TreatAsAtomicUnit=on
  If Action Subsystem4 : Subsystem  TreatAsAtomicUnit=on
  If Action Subsystem5 : Subsystem  TreatAsAtomicUnit=on
  If1 : If
  If2 : If  IfExpression=u1 == 0
  Merge : Merge
  Merge1 : Merge
  Merge2 : Merge
  Product : Product  Inputs=3
  Product5 : Product
  Relational Operator : RelationalOperator  OutDataTypeStr=boolean  RndMeth=Simplest
  P Flexor : Outport
  wires:
  If Action Subsystem3/1(Out1) -> Merge1/2
  Merge1/1 -> Generator PF/3, Relational Operator/1  "P Flexor"
  Constant1/1 -> If Action Subsystem1/1(In1)
  If1/1 -> If Action Subsystem2/Action
  If/1 -> If Action Subsystem/Action
  Function Caller4/1 -> Product/1
  Product/1 -> Generator PF/1, Relational Operator/2
  Merge/1 -> If1/1, If Action Subsystem2/1(In1)  "P Extenasor"
  If Action Subsystem/1(Out1) -> Merge/1
  If/2 -> If Action Subsystem1/Action
  If Action Subsystem1/1(Out1) -> Merge/2
  If1/2 -> If Action Subsystem3/Action
  Constant2/1 -> If Action Subsystem3/1(In1)
  Generator PF/1 -> P Flexor/1  "P Flexor"
  If Action Subsystem2/1(Out1) -> Merge1/1
  Activation/1 -> If/1, Product/3
  "Force "/1 -> If Action Subsystem/1("Force ")
  Relational Operator/1 -> Generator PF/2
  Function Caller10/1 -> If Action Subsystem4/1(In1), Product5/1
  If2/1 -> If Action Subsystem4/Action
  Constant/1 -> Product5/2
  Product5/1 -> If Action Subsystem5/1(In1)
  If2/2 -> If Action Subsystem5/Action
  Merge2/1 -> Product/2
  If Action Subsystem4/1(Out1) -> Merge2/1
  If Action Subsystem5/1(Out1) -> Merge2/2
  ModelAge/1 -> If2/1

== system InteractiveArmModel_R2021a_v1/While Loop (Main Simulation Code)/Muscle Models/Extensor Muscle Mechanics/Integrate Act Change ==
  note: If activation is very small, just set to zero.
  IC : Inport
  In2 : Inport  Port=2
  Constant3 : Constant  Value=0  SampleTime=-1
  If Action Subsystem4 : Subsystem  TreatAsAtomicUnit=on
  If Action Subsystem5 : Subsystem  TreatAsAtomicUnit=on
  If2 : If  IfExpression=u1>0.001
  Integrate Activation Rate of Change : Subsystem
  Merge2 : Merge
  Saturation : Saturate  UpperLimit=1  LowerLimit=0
  Zero if Sim Not Running : Subsystem
  Activation : Outport
  wires:
  If2/2 -> If Action Subsystem5/Action
  If Action Subsystem4/1(Out1) -> Merge2/1
  Integrate Activation Rate of Change/1(Velocity) -> Zero if Sim Not Running/2(" ")
  If Action Subsystem5/1(Out1) -> Merge2/2
  Constant3/1 -> If Action Subsystem5/1("Activation ")
  Merge2/1 -> Saturation/1
  IC/1 -> Zero if Sim Not Running/1(IC)
  Zero if Sim Not Running/1("Activation ") -> If2/1, If Action Subsystem4/1("Activation ")
  If2/1 -> If Action Subsystem4/Action
  Saturation/1 -> Activation/1
  In2/1 -> Integrate Activation Rate of Change/1(In1)

== system InteractiveArmModel_R2021a_v1/While Loop (Main Simulation Code)/Muscle Models/Extensor Muscle Mechanics/Reset ==
  1 : Inport
  " " : Inport  Port=2
  Display1 : Display
  Display2 : Display
  Display3 : Display
  If : If  IfExpression=u1 == 0  ShowElse=off
  If Action Subsystem : Subsystem  TreatAsAtomicUnit=on
  Subtract : Sum  Inputs=+-
  "Force " : Outport
  wires:
  1/1 -> If/1
  If/1 -> If Action Subsystem/Action
  Subtract/1 -> Display3/1, "Force "/1
  " "/1 -> Display1/1, Subtract/1, If Action Subsystem/1(In1)
  If Action Subsystem/1(Out1) -> Display2/1, Subtract/2

== system InteractiveArmModel_R2021a_v1/While Loop (Main Simulation Code)/Muscle Models/Extensor Muscle Mechanics/Subsystem ==
  dp/dt : Inport
  Add : Sum
  Delay : Delay  DelayLength=1  InitialCondition=0
  Delay1 : Delay  DelayLength=1  InitialCondition=0
  Digital Clock : DigitalClock  SampleTime=-1
  Product : Product
  Subtract : Sum  Inputs=+-
  Force : Outport
  wires:
  dp/dt/1 -> Product/2
  Subtract/1 -> Product/1
  Product/1 -> Add/1
  Add/1 -> Delay/1
  Delay/1 -> Force/1, Add/2
  Digital Clock/1 -> Subtract/1, Delay1/1
  Delay1/1 -> Subtract/2

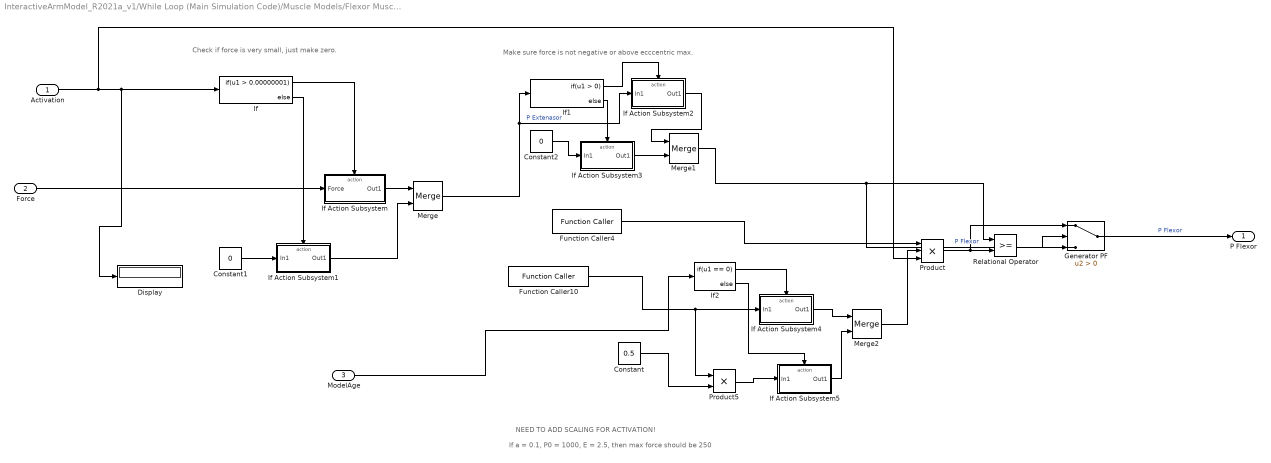
== system InteractiveArmModel_R2021a_v1/While Loop (Main Simulation Code)/Muscle Models/Flexor Muscle Mechanics/Bounds Checks ==
  note: If a = 0.1, P0 = 1000, E = 2.5, then max force should be 250
  note: NEED TO ADD SCALING FOR ACTIVATION!
  note: Check if force is very small, just make zero.
  note: Make sure force is not negative or above ecccentric max.
  Activation : Inport
  "Force " : Inport  Port=2
  ModelAge : Inport  Port=3
  Constant : Constant  Value=0.5
  Constant1 : Constant  Value=0
  Constant2 : Constant  Value=0
  Display : Display
  Function Caller10 : FunctionCaller  FunctionPrototype=y = Constants.P0F()  InputArgumentSpecifications=<Enter example>  OutputArgumentSpecifications=<Enter example>
  Function Caller4 : FunctionCaller  FunctionPrototype=y = Constants.EF()  InputArgumentSpecifications=<Enter example>  OutputArgumentSpecifications=<Enter example>
  Generator PF : Switch  Criteria=u2 > Threshold
  If : If  IfExpression=u1 > 0.00000001
  If Action Subsystem : Subsystem  TreatAsAtomicUnit=on
  If Action Subsystem1 : Subsystem  TreatAsAtomicUnit=on
  If Action Subsystem2 : Subsystem  TreatAsAtomicUnit=on
  If Action Subsystem3 : Subsystem  TreatAsAtomicUnit=on
  If Action Subsystem4 : Subsystem  TreatAsAtomicUnit=on
  If Action Subsystem5 : Subsystem  TreatAsAtomicUnit=on
  If1 : If
  If2 : If  IfExpression=u1 == 0
  Merge : Merge
  Merge1 : Merge
  Merge2 : Merge
  Product : Product  Inputs=3
  Product5 : Product
  Relational Operator : RelationalOperator  OutDataTypeStr=boolean  RndMeth=Simplest
  P Flexor : Outport
  wires:
  If Action Subsystem3/1(Out1) -> Merge1/2
  Merge1/1 -> Generator PF/3, Relational Operator/1  "P Flexor"
  Constant1/1 -> If Action Subsystem1/1(In1)
  If1/1 -> If Action Subsystem2/Action
  If/1 -> If Action Subsystem/Action
  Function Caller4/1 -> Product/1
  Product/1 -> Generator PF/1, Relational Operator/2
  Merge/1 -> If1/1, If Action Subsystem2/1(In1)  "P Extenasor"
  If Action Subsystem/1(Out1) -> Merge/1
  If/2 -> If Action Subsystem1/Action
  If Action Subsystem1/1(Out1) -> Merge/2
  If1/2 -> If Action Subsystem3/Action
  Constant2/1 -> If Action Subsystem3/1(In1)
  Generator PF/1 -> P Flexor/1  "P Flexor"
  If Action Subsystem2/1(Out1) -> Merge1/1
  Activation/1 -> Display/1, If/1, Product/3
  Relational Operator/1 -> Generator PF/2
  Function Caller10/1 -> If Action Subsystem4/1(In1), Product5/1
  If2/1 -> If Action Subsystem4/Action
  Constant/1 -> Product5/2
  Product5/1 -> If Action Subsystem5/1(In1)
  If2/2 -> If Action Subsystem5/Action
  Merge2/1 -> Product/2
  If Action Subsystem4/1(Out1) -> Merge2/1
  If Action Subsystem5/1(Out1) -> Merge2/2
  ModelAge/1 -> If2/1
  "Force "/1 -> If Action Subsystem/1("Force ")

== system InteractiveArmModel_R2021a_v1/While Loop (Main Simulation Code)/Muscle Models/Flexor Muscle Mechanics/Integrate Act Change ==
  note: If activation is very small, just set to zero.
  IC : Inport
  In2 : Inport  Port=2
  Constant3 : Constant  Value=0  SampleTime=-1
  If Action Subsystem4 : Subsystem  TreatAsAtomicUnit=on
  If Action Subsystem5 : Subsystem  TreatAsAtomicUnit=on
  If2 : If  IfExpression=u1>0.001
  Integrate Activation Rate of Change : Subsystem
  Merge2 : Merge
  Saturation : Saturate  UpperLimit=1  LowerLimit=0
  Zero if Sim Not Running : Subsystem
  Out1 : Outport
  wires:
  Constant3/1 -> If Action Subsystem5/1("Activation ")
  Zero if Sim Not Running/1("Activation ") -> If2/1, If Action Subsystem4/1("Activation ")
  Integrate Activation Rate of Change/1(Velocity) -> Zero if Sim Not Running/2(" ")
  If Action Subsystem5/1(Out1) -> Merge2/2
  If2/2 -> If Action Subsystem5/Action
  If Action Subsystem4/1(Out1) -> Merge2/1
  If2/1 -> If Action Subsystem4/Action
  Merge2/1 -> Saturation/1
  IC/1 -> Zero if Sim Not Running/1(IC)
  Saturation/1 -> Out1/1
  In2/1 -> Integrate Activation Rate of Change/1(In1)

== system InteractiveArmModel_R2021a_v1/While Loop (Main Simulation Code)/Muscle Models/Flexor Muscle Mechanics/Integrater ==
  In1 : Inport
  Add : Sum
  Delay : Delay  DelayLength=1  InitialCondition=0
  Delay1 : Delay  DelayLength=1  InitialCondition=0
  Digital Clock : DigitalClock  SampleTime=-1
  Product : Product
  Subtract : Sum  Inputs=+-
  1 : Outport
  wires:
  In1/1 -> Product/2
  Subtract/1 -> Product/1
  Product/1 -> Add/1
  Add/1 -> Delay/1
  Delay/1 -> 1/1, Add/2
  Digital Clock/1 -> Subtract/1, Delay1/1
  Delay1/1 -> Subtract/2

== system InteractiveArmModel_R2021a_v1/While Loop (Main Simulation Code)/Muscle Models/Flexor Muscle Mechanics/Reset ==
  1 : Inport
  " " : Inport  Port=2
  If : If  IfExpression=u1 == 0  ShowElse=off
  If Action Subsystem : Subsystem  TreatAsAtomicUnit=on
  Subtract : Sum  Inputs=+-
  "Force " : Outport
  wires:
  1/1 -> If/1
  If/1 -> If Action Subsystem/Action
  Subtract/1 -> "Force "/1
  " "/1 -> If Action Subsystem/1(In1), Subtract/1
  If Action Subsystem/1(Out1) -> Subtract/2

== system InteractiveArmModel_R2021a_v1/While Loop (Main Simulation Code)/Passive External Torques/Passive torque/If Action Subsystem1 ==
  In1 : Inport
  Action Port : ActionPort  ActionPortLabel=elseif(u1 < 5)
  Out1 : Outport
  wires:
  In1/1 -> Out1/1

== system InteractiveArmModel_R2021a_v1/While Loop (Main Simulation Code)/Passive External Torques/Passive torque/If Action Subsystem8 ==
  In1 : Inport
  Action Port : ActionPort  ActionPortLabel=if(u1 > 175)
  Out1 : Outport
  wires:
  In1/1 -> Out1/1

== system InteractiveArmModel_R2021a_v1/While Loop (Main Simulation Code)/Passive External Torques/Passive torque/If Action Subsystem9 ==
  In1 : Inport
  Action Port : ActionPort  ActionPortLabel=else
  Out1 : Outport
  wires:
  In1/1 -> Out1/1

== system InteractiveArmModel_R2021a_v1/While Loop (Main Simulation Code)/Muscle Models/Extensor Muscle Mechanics/Bounds Checks/If Action Subsystem ==
  "Force " : Inport
  Action Port : ActionPort  ActionPortLabel=if(u1 > 0.00000001)
  Out1 : Outport
  wires:
  "Force "/1 -> Out1/1

== system InteractiveArmModel_R2021a_v1/While Loop (Main Simulation Code)/Muscle Models/Extensor Muscle Mechanics/Bounds Checks/If Action Subsystem1 ==
  In1 : Inport
  Action Port : ActionPort  ActionPortLabel=else
  Out1 : Outport
  wires:
  In1/1 -> Out1/1

== system InteractiveArmModel_R2021a_v1/While Loop (Main Simulation Code)/Muscle Models/Extensor Muscle Mechanics/Bounds Checks/If Action Subsystem2 ==
  In1 : Inport
  Action Port : ActionPort  ActionPortLabel=if(u1 > 0)
  Out1 : Outport
  wires:
  In1/1 -> Out1/1

== system InteractiveArmModel_R2021a_v1/While Loop (Main Simulation Code)/Muscle Models/Extensor Muscle Mechanics/Bounds Checks/If Action Subsystem3 ==
  In1 : Inport
  Action Port : ActionPort  ActionPortLabel=else
  Out1 : Outport
  wires:
  In1/1 -> Out1/1

== system InteractiveArmModel_R2021a_v1/While Loop (Main Simulation Code)/Muscle Models/Extensor Muscle Mechanics/Bounds Checks/If Action Subsystem4 ==
  In1 : Inport
  Action Port : ActionPort  ActionPortLabel=if(u1 == 0)
  Out1 : Outport
  wires:
  In1/1 -> Out1/1

== system InteractiveArmModel_R2021a_v1/While Loop (Main Simulation Code)/Muscle Models/Extensor Muscle Mechanics/Bounds Checks/If Action Subsystem5 ==
  In1 : Inport
  Action Port : ActionPort  ActionPortLabel=else
  Out1 : Outport
  wires:
  In1/1 -> Out1/1

== system InteractiveArmModel_R2021a_v1/While Loop (Main Simulation Code)/Muscle Models/Extensor Muscle Mechanics/Integrate Act Change/If Action Subsystem4 ==
  "Activation " : Inport
  Action Port : ActionPort  ActionPortLabel=if(u1>0.001)
  Out1 : Outport
  wires:
  "Activation "/1 -> Out1/1

== system InteractiveArmModel_R2021a_v1/While Loop (Main Simulation Code)/Muscle Models/Extensor Muscle Mechanics/Integrate Act Change/If Action Subsystem5 ==
  "Activation " : Inport
  Action Port : ActionPort  ActionPortLabel=else
  Out1 : Outport
  wires:
  "Activation "/1 -> Out1/1

== system InteractiveArmModel_R2021a_v1/While Loop (Main Simulation Code)/Muscle Models/Extensor Muscle Mechanics/Integrate Act Change/Integrate Activation Rate of Change ==
  In1 : Inport
  Add : Sum
  Delay : Delay  DelayLength=1  InitialCondition=0
  Delay1 : Delay  DelayLength=1  InitialCondition=0
  Digital Clock : DigitalClock  SampleTime=-1
  Product : Product
  Subtract : Sum  Inputs=+-
  Velocity : Outport
  wires:
  In1/1 -> Product/2
  Subtract/1 -> Product/1
  Product/1 -> Add/1
  Add/1 -> Delay/1
  Delay/1 -> Velocity/1, Add/2
  Digital Clock/1 -> Subtract/1, Delay1/1
  Delay1/1 -> Subtract/2

== system InteractiveArmModel_R2021a_v1/While Loop (Main Simulation Code)/Muscle Models/Extensor Muscle Mechanics/Integrate Act Change/Zero if Sim Not Running ==
  note: If simulation not "Active", keep activation zero.
  IC : Inport
  " " : Inport  Port=2
  Constant : Constant  Value=0
  If : If  IfExpression=u1 == 0
  If Action Subsystem : Subsystem  TreatAsAtomicUnit=on
  If Action Subsystem7 : Subsystem  TreatAsAtomicUnit=on
  Merge2 : Merge
  "Activation " : Outport
  wires:
  IC/1 -> If/1
  If/1 -> If Action Subsystem/Action
  Merge2/1 -> "Activation "/1
  Constant/1 -> If Action Subsystem/1(In1)
  If/2 -> If Action Subsystem7/Action
  " "/1 -> If Action Subsystem7/1(" ")  "Activation"
  If Action Subsystem/1(Out1) -> Merge2/1
  If Action Subsystem7/1(Out1) -> Merge2/2

== system InteractiveArmModel_R2021a_v1/While Loop (Main Simulation Code)/Muscle Models/Extensor Muscle Mechanics/Reset/If Action Subsystem ==
  In1 : Inport
  Action Port : ActionPort  ActionPortLabel=if(u1 == 0)
  Out1 : Outport
  wires:
  In1/1 -> Out1/1

== system InteractiveArmModel_R2021a_v1/While Loop (Main Simulation Code)/Muscle Models/Flexor Muscle Mechanics/Bounds Checks/If Action Subsystem ==
  "Force " : Inport
  Action Port : ActionPort  ActionPortLabel=if(u1 > 0.00000001)
  Out1 : Outport
  wires:
  "Force "/1 -> Out1/1

== system InteractiveArmModel_R2021a_v1/While Loop (Main Simulation Code)/Muscle Models/Flexor Muscle Mechanics/Bounds Checks/If Action Subsystem1 ==
  In1 : Inport
  Action Port : ActionPort  ActionPortLabel=else
  Out1 : Outport
  wires:
  In1/1 -> Out1/1

== system InteractiveArmModel_R2021a_v1/While Loop (Main Simulation Code)/Muscle Models/Flexor Muscle Mechanics/Bounds Checks/If Action Subsystem2 ==
  In1 : Inport
  Action Port : ActionPort  ActionPortLabel=if(u1 > 0)
  Out1 : Outport
  wires:
  In1/1 -> Out1/1

== system InteractiveArmModel_R2021a_v1/While Loop (Main Simulation Code)/Muscle Models/Flexor Muscle Mechanics/Bounds Checks/If Action Subsystem3 ==
  In1 : Inport
  Action Port : ActionPort  ActionPortLabel=else
  Out1 : Outport
  wires:
  In1/1 -> Out1/1

== system InteractiveArmModel_R2021a_v1/While Loop (Main Simulation Code)/Muscle Models/Flexor Muscle Mechanics/Bounds Checks/If Action Subsystem4 ==
  In1 : Inport
  Action Port : ActionPort  ActionPortLabel=if(u1 == 0)
  Out1 : Outport
  wires:
  In1/1 -> Out1/1

== system InteractiveArmModel_R2021a_v1/While Loop (Main Simulation Code)/Muscle Models/Flexor Muscle Mechanics/Bounds Checks/If Action Subsystem5 ==
  In1 : Inport
  Action Port : ActionPort  ActionPortLabel=else
  Out1 : Outport
  wires:
  In1/1 -> Out1/1

== system InteractiveArmModel_R2021a_v1/While Loop (Main Simulation Code)/Muscle Models/Flexor Muscle Mechanics/Integrate Act Change/If Action Subsystem4 ==
  "Activation " : Inport
  Action Port : ActionPort  ActionPortLabel=if(u1>0.001)
  Out1 : Outport
  wires:
  "Activation "/1 -> Out1/1

== system InteractiveArmModel_R2021a_v1/While Loop (Main Simulation Code)/Muscle Models/Flexor Muscle Mechanics/Integrate Act Change/If Action Subsystem5 ==
  "Activation " : Inport
  Action Port : ActionPort  ActionPortLabel=else
  Out1 : Outport
  wires:
  "Activation "/1 -> Out1/1

== system InteractiveArmModel_R2021a_v1/While Loop (Main Simulation Code)/Muscle Models/Flexor Muscle Mechanics/Integrate Act Change/Integrate Activation Rate of Change ==
  In1 : Inport
  Add : Sum
  Delay : Delay  DelayLength=1  InitialCondition=0
  Delay1 : Delay  DelayLength=1  InitialCondition=0
  Digital Clock : DigitalClock  SampleTime=-1
  Product : Product
  Subtract : Sum  Inputs=+-
  Velocity : Outport
  wires:
  In1/1 -> Product/2
  Subtract/1 -> Product/1
  Product/1 -> Add/1
  Add/1 -> Delay/1
  Delay/1 -> Velocity/1, Add/2
  Digital Clock/1 -> Subtract/1, Delay1/1
  Delay1/1 -> Subtract/2

== system InteractiveArmModel_R2021a_v1/While Loop (Main Simulation Code)/Muscle Models/Flexor Muscle Mechanics/Integrate Act Change/Zero if Sim Not Running ==
  note: If simulation not "Active", keep activation zero.
  IC : Inport
  " " : Inport  Port=2
  Constant : Constant  Value=0
  If : If  IfExpression=u1 == 0
  If Action Subsystem : Subsystem  TreatAsAtomicUnit=on
  If Action Subsystem7 : Subsystem  TreatAsAtomicUnit=on
  Merge2 : Merge
  "Activation " : Outport
  wires:
  IC/1 -> If/1
  If/1 -> If Action Subsystem/Action
  Merge2/1 -> "Activation "/1
  Constant/1 -> If Action Subsystem/1(In1)
  If/2 -> If Action Subsystem7/Action
  " "/1 -> If Action Subsystem7/1(" ")  "Activation"
  If Action Subsystem/1(Out1) -> Merge2/1
  If Action Subsystem7/1(Out1) -> Merge2/2

== system InteractiveArmModel_R2021a_v1/While Loop (Main Simulation Code)/Muscle Models/Flexor Muscle Mechanics/Reset/If Action Subsystem ==
  In1 : Inport
  Action Port : ActionPort  ActionPortLabel=if(u1 == 0)
  Out1 : Outport
  wires:
  In1/1 -> Out1/1

== system InteractiveArmModel_R2021a_v1/While Loop (Main Simulation Code)/Muscle Models/Extensor Muscle Mechanics/Integrate Act Change/Zero if Sim Not Running/If Action Subsystem ==
  In1 : Inport
  Action Port : ActionPort  ActionPortLabel=if(u1 == 0)
  Out1 : Outport
  wires:
  In1/1 -> Out1/1

== system InteractiveArmModel_R2021a_v1/While Loop (Main Simulation Code)/Muscle Models/Extensor Muscle Mechanics/Integrate Act Change/Zero if Sim Not Running/If Action Subsystem7 ==
  " " : Inport
  Action Port : ActionPort  ActionPortLabel=else
  Out1 : Outport
  wires:
  " "/1 -> Out1/1

== system InteractiveArmModel_R2021a_v1/While Loop (Main Simulation Code)/Muscle Models/Flexor Muscle Mechanics/Integrate Act Change/Zero if Sim Not Running/If Action Subsystem ==
  In1 : Inport
  Action Port : ActionPort  ActionPortLabel=if(u1 == 0)
  Out1 : Outport
  wires:
  In1/1 -> Out1/1

== system InteractiveArmModel_R2021a_v1/While Loop (Main Simulation Code)/Muscle Models/Flexor Muscle Mechanics/Integrate Act Change/Zero if Sim Not Running/If Action Subsystem7 ==
  " " : Inport
  Action Port : ActionPort  ActionPortLabel=else
  Out1 : Outport
  wires:
  " "/1 -> Out1/1
